simulink model "Microgrid_6DGs"  (R2024a)
settings: Solver=VariableStepAuto  StartTime=0.0  StopTime=10  RelTol=1e-3
values from neighbouring files (symbols this model uses):
  DG = cell(1, numOfDGs)    [evaluateDesigns.m]
  K = cell(1, numDGs)    [Centralized_Controller_For_DG.m]    (also in Centralized_Controller_For_DG_with_Constraints.m; ComputePassivityForDGs.m = sdpvar(1, 3, 'full'); GetPassivityForDGs.m = sdpvar(1, 3, 'full'); Global_Controller_Synthesis.m = cell(N, N))
  Line = cell(1, numOfLines)    [evaluateDesigns.m]
  numOfDGs = size(B_il,1)    [OptimizeMGparameters.m]    (also in OptimizepValsMethod1.m; centralizedCodesign.m; centralizedCodesignFeasibility.m; centralizedLocalControlDesign-Mohammad’s Laptop.m)
  V_ref = 48    [Global_Controller_Synthesis.m]
undefined symbols (not defined in the file or in its folder): change_reference, PlugIn, PlugOut, V_nom, V_ref1, V_ref2
libraries: spsSeriesRLCBranchLib x48, spsCurrentMeasurementLib x12, simulink x6, spsIdealSwitchLib x6, spsStairGeneratorLib x6, spsControlledCurrentSourceLib x6, spsDCVoltageSourceLib x6, spsDiodeLib x6, spsIGBTLib x6, spsVoltageMeasurementLib x6, spspowerguiLib x1
(part 2 of 2)

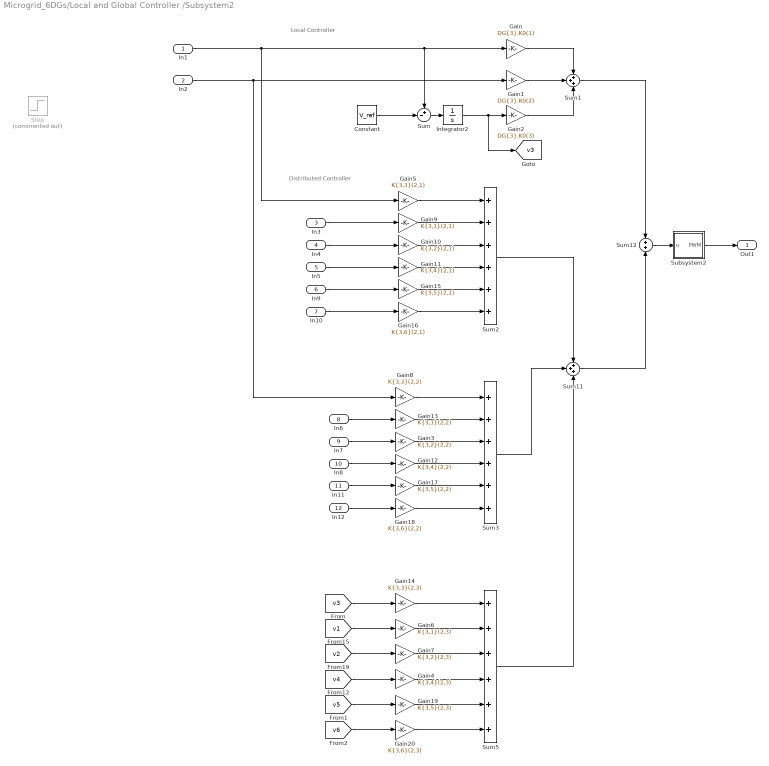
== system Microgrid_6DGs/Local and Global Controller /Subsystem2 ==
  note: Distributed Controller
  note: Local Controller
  In1 : Inport
  In2 : Inport  Port=2
  In3 : Inport  Port=3
  In4 : Inport  Port=4
  In5 : Inport  Port=5
  In9 : Inport  Port=6
  In10 : Inport  Port=7
  In6 : Inport  Port=8
  In7 : Inport  Port=9
  In8 : Inport  Port=10
  In11 : Inport  Port=11
  In12 : Inport  Port=12
  Constant : Constant  Value=V_ref
  Gain : Gain  Gain=DG{3}.K0(1)
  Gain1 : Gain  Gain=DG{3}.K0(2)
  Gain10 : Gain  Gain=K{3,2}(2,1)
  Gain11 : Gain  Gain=K{3,4}(2,1)
  Gain12 : Gain  Gain=K{3,4}(2,2)
  Gain13 : Gain  Gain=K{3,1}(2,2)
  Gain14 : Gain  Gain=K{3,3}(2,3)
  Gain15 : Gain  Gain=K{3,5}(2,1)
  Gain16 : Gain  Gain=K{3,6}(2,1)
  Gain17 : Gain  Gain=K{3,5}(2,2)
  Gain18 : Gain  Gain=K{3,6}(2,2)
  Gain19 : Gain  Gain=K{3,5}(2,3)
  Gain2 : Gain  Gain=DG{3}.K0(3)
  Gain20 : Gain  Gain=K{3,6}(2,3)
  Gain3 : Gain  Gain=K{3,2}(2,2)
  Gain4 : Gain  Gain=K{3,4}(2,3)
  Gain5 : Gain  Gain=K{3,3}(2,1)
  Gain6 : Gain  Gain=K{3,1}(2,3)
  Gain7 : Gain  Gain=K{3,2}(2,3)
  Gain8 : Gain  Gain=K{3,3}(2,2)
  Gain9 : Gain  Gain=K{3,1}(2,1)
  Integrator2 : Integrator
  Step : Step  Commented=on  Time=change_reference  Before=V_ref1  After=V_ref2  SampleTime=0
  Subsystem2 : Subsystem
      mask Display: disp('PWM')
  Sum : Sum  Inputs=+-|
  Sum1 : Sum  Inputs=+++
  Sum11 : Sum  Inputs=+++
  Sum12 : Sum  Inputs=+|+
  Sum2 : Sum  Inputs=++++++
  Sum3 : Sum  Inputs=++++++
  Sum5 : Sum  Inputs=++++++
  Out1 : Outport
  tag scope: v3=global
  wires:
  Gain/1 -> Sum1/1
  Gain1/1 -> Sum1/2
  Sum1/1 -> Sum12/1
  Gain6/1 -> Sum5/2
  Gain13/1 -> Sum3/2
  Gain12/1 -> Sum3/4
  Gain7/1 -> Sum5/3
  Gain5/1 -> Sum2/1
  Gain3/1 -> Sum3/3
  Sum11/1 -> Sum12/2
  Gain4/1 -> Sum5/4
  In4/1 -> Gain10/1
  [v2] -> Gain7/1
  In3/1 -> Gain9/1
  [v1] -> Gain6/1
  In6/1 -> Gain13/1
  [v4] -> Gain4/1
  In8/1 -> Gain12/1
  Gain10/1 -> Sum2/3
  In7/1 -> Gain3/1
  In5/1 -> Gain11/1
  Gain14/1 -> Sum5/1
  Gain11/1 -> Sum2/4
  Gain9/1 -> Sum2/2
  Gain8/1 -> Sum3/1
  [v3] -> Gain14/1
  Sum2/1 -> Sum11/1
  Sum3/1 -> Sum11/2
  Sum5/1 -> Sum11/3
  Sum/1 -> Integrator2/1
  In2/1 -> Gain1/1, Gain8/1
  In1/1 -> Gain/1, Sum/1, Gain5/1
  Sum12/1 -> Subsystem2/1(u)
  Subsystem2/1(PWM) -> Out1/1
  Constant/1 -> Sum/2
  Gain15/1 -> Sum2/5
  Gain16/1 -> Sum2/6
  In9/1 -> Gain15/1
  In10/1 -> Gain16/1
  Gain17/1 -> Sum3/5
  In11/1 -> Gain17/1
  Gain18/1 -> Sum3/6
  In12/1 -> Gain18/1
  Gain19/1 -> Sum5/5
  Gain20/1 -> Sum5/6
  [v5] -> Gain19/1
  [v6] -> Gain20/1
  Gain2/1 -> Sum1/3
  Integrator2/1 -> [v3], Gain2/1

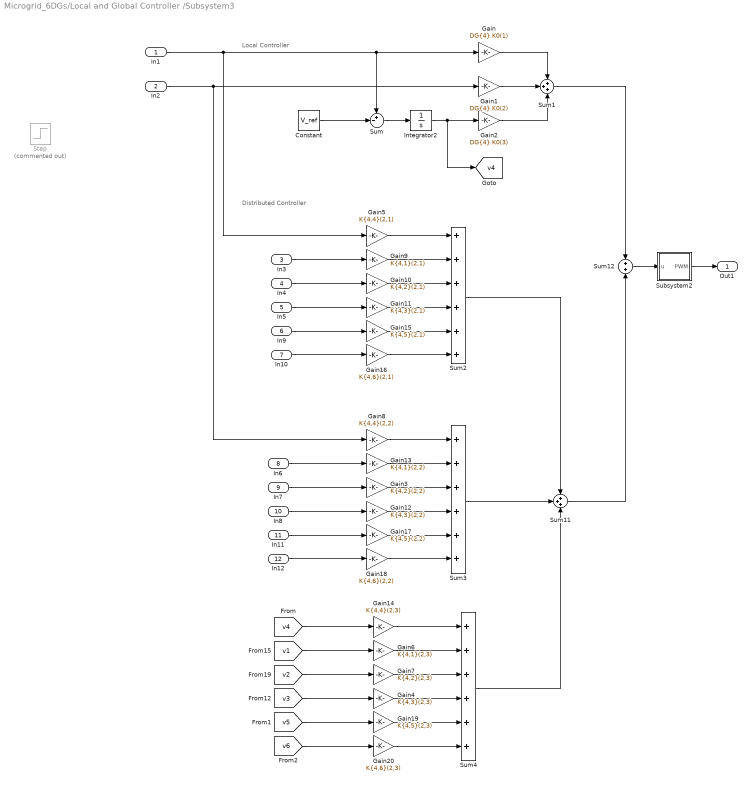
== system Microgrid_6DGs/Local and Global Controller /Subsystem3 ==
  note: Distributed Controller
  note: Local Controller
  In1 : Inport
  In2 : Inport  Port=2
  In3 : Inport  Port=3
  In4 : Inport  Port=4
  In5 : Inport  Port=5
  In9 : Inport  Port=6
  In10 : Inport  Port=7
  In6 : Inport  Port=8
  In7 : Inport  Port=9
  In8 : Inport  Port=10
  In11 : Inport  Port=11
  In12 : Inport  Port=12
  Constant : Constant  Value=V_ref
  Gain : Gain  Gain=DG{4}.K0(1)
  Gain1 : Gain  Gain=DG{4}.K0(2)
  Gain10 : Gain  Gain=K{4,2}(2,1)
  Gain11 : Gain  Gain=K{4,3}(2,1)
  Gain12 : Gain  Gain=K{4,3}(2,2)
  Gain13 : Gain  Gain=K{4,1}(2,2)
  Gain14 : Gain  Gain=K{4,4}(2,3)
  Gain15 : Gain  Gain=K{4,5}(2,1)
  Gain16 : Gain  Gain=K{4,6}(2,1)
  Gain17 : Gain  Gain=K{4,5}(2,2)
  Gain18 : Gain  Gain=K{4,6}(2,2)
  Gain19 : Gain  Gain=K{4,5}(2,3)
  Gain2 : Gain  Gain=DG{4}.K0(3)
  Gain20 : Gain  Gain=K{4,6}(2,3)
  Gain3 : Gain  Gain=K{4,2}(2,2)
  Gain4 : Gain  Gain=K{4,3}(2,3)
  Gain5 : Gain  Gain=K{4,4}(2,1)
  Gain6 : Gain  Gain=K{4,1}(2,3)
  Gain7 : Gain  Gain=K{4,2}(2,3)
  Gain8 : Gain  Gain=K{4,4}(2,2)
  Gain9 : Gain  Gain=K{4,1}(2,1)
  Integrator2 : Integrator
  Step : Step  Commented=on  Time=change_reference  Before=V_ref1  After=V_ref2  SampleTime=0
  Subsystem2 : Subsystem
      mask Display: disp('PWM')
  Sum : Sum  Inputs=+-|
  Sum1 : Sum  Inputs=+++
  Sum11 : Sum  Inputs=+++
  Sum12 : Sum  Inputs=+|+
  Sum2 : Sum  Inputs=++++++
  Sum3 : Sum  Inputs=++++++
  Sum4 : Sum  Inputs=++++++
  Out1 : Outport
  tag scope: v4=global
  wires:
  Sum1/1 -> Sum12/1
  Gain1/1 -> Sum1/2
  Gain/1 -> Sum1/1
  Gain6/1 -> Sum4/2
  Gain13/1 -> Sum3/2
  Gain12/1 -> Sum3/4
  Gain7/1 -> Sum4/3
  Gain5/1 -> Sum2/1
  Gain3/1 -> Sum3/3
  Sum11/1 -> Sum12/2
  Gain4/1 -> Sum4/4
  In4/1 -> Gain10/1
  [v2] -> Gain7/1
  In3/1 -> Gain9/1
  [v1] -> Gain6/1
  In6/1 -> Gain13/1
  [v3] -> Gain4/1
  In8/1 -> Gain12/1
  Gain10/1 -> Sum2/3
  In7/1 -> Gain3/1
  In5/1 -> Gain11/1
  Gain14/1 -> Sum4/1
  Gain11/1 -> Sum2/4
  Gain9/1 -> Sum2/2
  Gain8/1 -> Sum3/1
  [v4] -> Gain14/1
  Sum2/1 -> Sum11/1
  Sum3/1 -> Sum11/2
  Sum4/1 -> Sum11/3
  Sum/1 -> Integrator2/1
  In2/1 -> Gain1/1, Gain8/1
  In1/1 -> Gain/1, Sum/1, Gain5/1
  Sum12/1 -> Subsystem2/1(u)
  Subsystem2/1(PWM) -> Out1/1
  Constant/1 -> Sum/2
  Gain15/1 -> Sum2/5
  In9/1 -> Gain15/1
  Gain16/1 -> Sum2/6
  In10/1 -> Gain16/1
  Gain17/1 -> Sum3/5
  Gain18/1 -> Sum3/6
  In11/1 -> Gain17/1
  In12/1 -> Gain18/1
  Gain19/1 -> Sum4/5
  [v5] -> Gain19/1
  Gain20/1 -> Sum4/6
  [v6] -> Gain20/1
  Gain2/1 -> Sum1/3
  Integrator2/1 -> [v4], Gain2/1

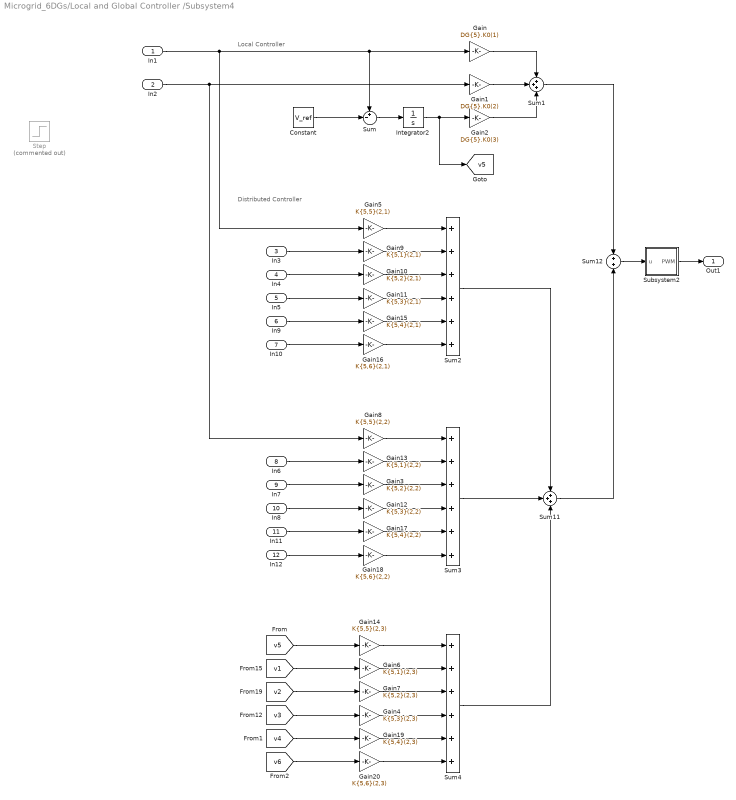
== system Microgrid_6DGs/Local and Global Controller /Subsystem4 ==
  note: Local Controller
  note: Distributed Controller
  In1 : Inport
  In2 : Inport  Port=2
  In3 : Inport  Port=3
  In4 : Inport  Port=4
  In5 : Inport  Port=5
  In9 : Inport  Port=6
  In10 : Inport  Port=7
  In6 : Inport  Port=8
  In7 : Inport  Port=9
  In8 : Inport  Port=10
  In11 : Inport  Port=11
  In12 : Inport  Port=12
  Constant : Constant  Value=V_ref
  Gain : Gain  Gain=DG{5}.K0(1)
  Gain1 : Gain  Gain=DG{5}.K0(2)
  Gain10 : Gain  Gain=K{5,2}(2,1)
  Gain11 : Gain  Gain=K{5,3}(2,1)
  Gain12 : Gain  Gain=K{5,3}(2,2)
  Gain13 : Gain  Gain=K{5,1}(2,2)
  Gain14 : Gain  Gain=K{5,5}(2,3)
  Gain15 : Gain  Gain=K{5,4}(2,1)
  Gain16 : Gain  Gain=K{5,6}(2,1)
  Gain17 : Gain  Gain=K{5,4}(2,2)
  Gain18 : Gain  Gain=K{5,6}(2,2)
  Gain19 : Gain  Gain=K{5,4}(2,3)
  Gain2 : Gain  Gain=DG{5}.K0(3)
  Gain20 : Gain  Gain=K{5,6}(2,3)
  Gain3 : Gain  Gain=K{5,2}(2,2)
  Gain4 : Gain  Gain=K{5,3}(2,3)
  Gain5 : Gain  Gain=K{5,5}(2,1)
  Gain6 : Gain  Gain=K{5,1}(2,3)
  Gain7 : Gain  Gain=K{5,2}(2,3)
  Gain8 : Gain  Gain=K{5,5}(2,2)
  Gain9 : Gain  Gain=K{5,1}(2,1)
  Integrator2 : Integrator
  Step : Step  Commented=on  Time=change_reference  Before=V_ref1  After=V_ref2  SampleTime=0
  Subsystem2 : Subsystem
      mask Display: disp('PWM')
  Sum : Sum  Inputs=+-|
  Sum1 : Sum  Inputs=+++
  Sum11 : Sum  Inputs=+++
  Sum12 : Sum  Inputs=+|+
  Sum2 : Sum  Inputs=++++++
  Sum3 : Sum  Inputs=++++++
  Sum4 : Sum  Inputs=++++++
  Out1 : Outport
  tag scope: v5=global
  wires:
  Constant/1 -> Sum/2
  Subsystem2/1(PWM) -> Out1/1
  Sum12/1 -> Subsystem2/1(u)
  In1/1 -> Gain5/1, Sum/1, Gain/1
  In2/1 -> Gain8/1, Gain1/1
  Sum/1 -> Integrator2/1
  Sum4/1 -> Sum11/3
  Sum3/1 -> Sum11/2
  Sum2/1 -> Sum11/1
  [v5] -> Gain14/1
  Gain8/1 -> Sum3/1
  Gain9/1 -> Sum2/2
  Gain11/1 -> Sum2/4
  Gain14/1 -> Sum4/1
  In5/1 -> Gain11/1
  In7/1 -> Gain3/1
  Gain10/1 -> Sum2/3
  In8/1 -> Gain12/1
  [v3] -> Gain4/1
  In6/1 -> Gain13/1
  [v1] -> Gain6/1
  In3/1 -> Gain9/1
  [v2] -> Gain7/1
  In4/1 -> Gain10/1
  Gain4/1 -> Sum4/4
  Sum11/1 -> Sum12/2
  Gain3/1 -> Sum3/3
  Gain5/1 -> Sum2/1
  Gain7/1 -> Sum4/3
  Gain12/1 -> Sum3/4
  Gain13/1 -> Sum3/2
  Gain6/1 -> Sum4/2
  Gain/1 -> Sum1/1
  Gain1/1 -> Sum1/2
  Sum1/1 -> Sum12/1
  Gain15/1 -> Sum2/5
  Gain16/1 -> Sum2/6
  In9/1 -> Gain15/1
  In10/1 -> Gain16/1
  Gain17/1 -> Sum3/5
  In11/1 -> Gain17/1
  Gain18/1 -> Sum3/6
  In12/1 -> Gain18/1
  Gain19/1 -> Sum4/5
  Gain20/1 -> Sum4/6
  [v4] -> Gain19/1
  [v6] -> Gain20/1
  Gain2/1 -> Sum1/3
  Integrator2/1 -> Gain2/1, [v5]

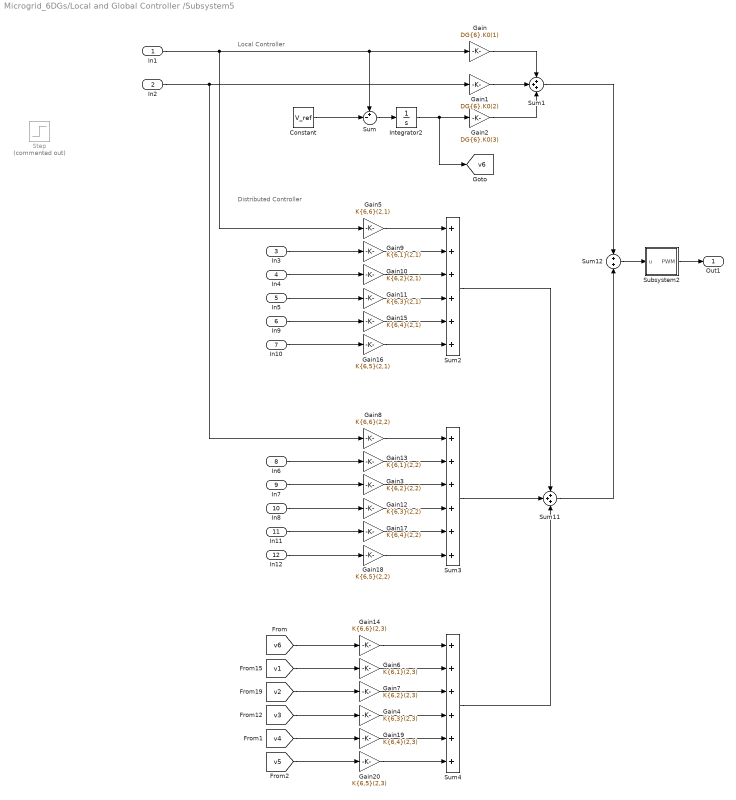
== system Microgrid_6DGs/Local and Global Controller /Subsystem5 ==
  note: Distributed Controller
  note: Local Controller
  In1 : Inport
  In2 : Inport  Port=2
  In3 : Inport  Port=3
  In4 : Inport  Port=4
  In5 : Inport  Port=5
  In9 : Inport  Port=6
  In10 : Inport  Port=7
  In6 : Inport  Port=8
  In7 : Inport  Port=9
  In8 : Inport  Port=10
  In11 : Inport  Port=11
  In12 : Inport  Port=12
  Constant : Constant  Value=V_ref
  Gain : Gain  Gain=DG{6}.K0(1)
  Gain1 : Gain  Gain=DG{6}.K0(2)
  Gain10 : Gain  Gain=K{6,2}(2,1)
  Gain11 : Gain  Gain=K{6,3}(2,1)
  Gain12 : Gain  Gain=K{6,3}(2,2)
  Gain13 : Gain  Gain=K{6,1}(2,2)
  Gain14 : Gain  Gain=K{6,6}(2,3)
  Gain15 : Gain  Gain=K{6,4}(2,1)
  Gain16 : Gain  Gain=K{6,5}(2,1)
  Gain17 : Gain  Gain=K{6,4}(2,2)
  Gain18 : Gain  Gain=K{6,5}(2,2)
  Gain19 : Gain  Gain=K{6,4}(2,3)
  Gain2 : Gain  Gain=DG{6}.K0(3)
  Gain20 : Gain  Gain=K{6,5}(2,3)
  Gain3 : Gain  Gain=K{6,2}(2,2)
  Gain4 : Gain  Gain=K{6,3}(2,3)
  Gain5 : Gain  Gain=K{6,6}(2,1)
  Gain6 : Gain  Gain=K{6,1}(2,3)
  Gain7 : Gain  Gain=K{6,2}(2,3)
  Gain8 : Gain  Gain=K{6,6}(2,2)
  Gain9 : Gain  Gain=K{6,1}(2,1)
  Integrator2 : Integrator
  Step : Step  Commented=on  Time=change_reference  Before=V_ref1  After=V_ref2  SampleTime=0
  Subsystem2 : Subsystem
      mask Display: disp('PWM')
  Sum : Sum  Inputs=+-|
  Sum1 : Sum  Inputs=+++
  Sum11 : Sum  Inputs=+++
  Sum12 : Sum  Inputs=+|+
  Sum2 : Sum  Inputs=++++++
  Sum3 : Sum  Inputs=++++++
  Sum4 : Sum  Inputs=++++++
  Out1 : Outport
  tag scope: v6=global
  wires:
  [v5] -> Gain20/1
  [v4] -> Gain19/1
  Gain20/1 -> Sum4/6
  Gain19/1 -> Sum4/5
  In12/1 -> Gain18/1
  Gain18/1 -> Sum3/6
  In11/1 -> Gain17/1
  Gain17/1 -> Sum3/5
  In10/1 -> Gain16/1
  In9/1 -> Gain15/1
  Gain16/1 -> Sum2/6
  Gain15/1 -> Sum2/5
  Sum1/1 -> Sum12/1
  Gain1/1 -> Sum1/2
  Gain/1 -> Sum1/1
  Gain6/1 -> Sum4/2
  Gain13/1 -> Sum3/2
  Gain12/1 -> Sum3/4
  Gain7/1 -> Sum4/3
  Gain5/1 -> Sum2/1
  Gain3/1 -> Sum3/3
  Sum11/1 -> Sum12/2
  Gain4/1 -> Sum4/4
  In4/1 -> Gain10/1
  [v2] -> Gain7/1
  In3/1 -> Gain9/1
  [v1] -> Gain6/1
  In6/1 -> Gain13/1
  [v3] -> Gain4/1
  In8/1 -> Gain12/1
  Gain10/1 -> Sum2/3
  In7/1 -> Gain3/1
  In5/1 -> Gain11/1
  Gain14/1 -> Sum4/1
  Gain11/1 -> Sum2/4
  Gain9/1 -> Sum2/2
  Gain8/1 -> Sum3/1
  [v6] -> Gain14/1
  Sum2/1 -> Sum11/1
  Sum3/1 -> Sum11/2
  Sum4/1 -> Sum11/3
  Sum/1 -> Integrator2/1
  In2/1 -> Gain1/1, Gain8/1
  In1/1 -> Gain/1, Sum/1, Gain5/1
  Sum12/1 -> Subsystem2/1(u)
  Subsystem2/1(PWM) -> Out1/1
  Constant/1 -> Sum/2
  Gain2/1 -> Sum1/3
  Integrator2/1 -> [v6], Gain2/1

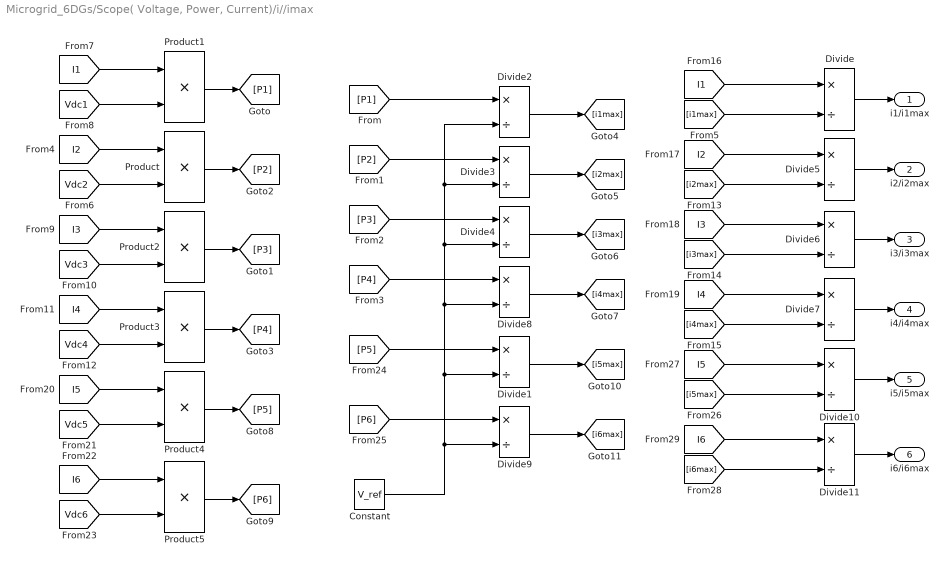
== system Microgrid_6DGs/Scope( Voltage, Power, Current)/i//imax ==
  Constant : Constant  Value=V_ref
  Divide{,1..11} (12 alike) : Product  Inputs=*/
  Product{,1..5} (6 alike) : Product
  i1/i1max : Outport  VectorParamsAs1DForOutWhenUnconnected=off
  i2/i2max : Outport  Port=2  VectorParamsAs1DForOutWhenUnconnected=off
  i3/i3max : Outport  Port=3  VectorParamsAs1DForOutWhenUnconnected=off
  i4/i4max : Outport  Port=4  VectorParamsAs1DForOutWhenUnconnected=off
  i5/i5max : Outport  Port=5  VectorParamsAs1DForOutWhenUnconnected=off
  i6/i6max : Outport  Port=6  VectorParamsAs1DForOutWhenUnconnected=off
  wires:
  Divide/1 -> i1/i1max/1
  Divide5/1 -> i2/i2max/1
  Divide6/1 -> i3/i3max/1
  Divide7/1 -> i4/i4max/1
  [Vdc3] -> Product2/2
  [Vdc1] -> Product1/2
  [Vdc2] -> Product/2
  [I1] -> Product1/1
  [I2] -> Product/1
  [Vdc4] -> Product3/2
  [I4] -> Product3/1
  [I3] -> Product2/1
  Product1/1 -> [P1]
  Product2/1 -> [P3]
  Product/1 -> [P2]
  Product3/1 -> [P4]
  [P1] -> Divide2/1
  [P2] -> Divide3/1
  [P3] -> Divide4/1
  [P4] -> Divide8/1
  Constant/1 -> Divide9/2, Divide1/2, Divide8/2, Divide4/2, Divide3/2, Divide2/2
  Divide8/1 -> [i4max]
  Divide4/1 -> [i3max]
  Divide3/1 -> [i2max]
  Divide2/1 -> [i1max]
  [i1max] -> Divide/2
  [i2max] -> Divide5/2
  [i3max] -> Divide6/2
  [i4max] -> Divide7/2
  [I1] -> Divide/1
  [I2] -> Divide5/1
  [I3] -> Divide6/1
  [I4] -> Divide7/1
  Product4/1 -> [P5]
  [I5] -> Product4/1
  [Vdc5] -> Product4/2
  [Vdc6] -> Product5/2
  [I6] -> Product5/1
  Product5/1 -> [P6]
  [P5] -> Divide1/1
  [P6] -> Divide9/1
  Divide1/1 -> [i5max]
  Divide9/1 -> [i6max]
  [I5] -> Divide10/1
  [i5max] -> Divide10/2
  Divide10/1 -> i5/i5max/1
  Divide11/1 -> i6/i6max/1
  [i6max] -> Divide11/2
  [I6] -> Divide11/1

== system Microgrid_6DGs/Subsystem/Breaker3 ==
  Ideal Switch : spsIdealSwitchLib/Ideal Switch  Ron=0.001  Lon=0  IC=0  Rs=1e5  Cs=inf  Measurements=on
  Stair Generator : spsStairGeneratorLib/Stair Generator  t=[0,PlugOut,PlugIn]  e=[1, 0, 1]  Ts=0
  DG3 : PMIOPort  Side=Left
  + : PMIOPort  Port=2  Side=Right
  wires:
  Stair Generator/1 -> Ideal Switch/1
  connections:
  Ideal Switch/LConn1 -- DG3/RConn1
  Ideal Switch/RConn1 -- +/RConn1

== system Microgrid_6DGs/Subsystem1/Breaker1 ==
  Ideal Switch : spsIdealSwitchLib/Ideal Switch  Ron=0.001  Lon=0  IC=0  Rs=1e5  Cs=inf  Measurements=on
  Stair Generator : spsStairGeneratorLib/Stair Generator  t=[0,PlugOut,PlugIn]  e=[1, 0, 1]  Ts=0
  DG1 : PMIOPort  Side=Left
  + : PMIOPort  Port=2  Side=Right
  wires:
  Stair Generator/1 -> Ideal Switch/1
  connections:
  Ideal Switch/LConn1 -- DG1/RConn1
  Ideal Switch/RConn1 -- +/RConn1

== system Microgrid_6DGs/Subsystem2/Breaker1 ==
  Ideal Switch : spsIdealSwitchLib/Ideal Switch  Ron=0.001  Lon=0  IC=0  Rs=1e5  Cs=inf  Measurements=on
  Stair Generator : spsStairGeneratorLib/Stair Generator  t=[0,PlugOut,PlugIn]  e=[1, 0, 1]  Ts=0
  DG1 : PMIOPort  Side=Left
  + : PMIOPort  Port=2  Side=Right
  wires:
  Stair Generator/1 -> Ideal Switch/1
  connections:
  Ideal Switch/RConn1 -- +/RConn1
  Ideal Switch/LConn1 -- DG1/RConn1

== system Microgrid_6DGs/Subsystem4/Breaker1 ==
  Ideal Switch : spsIdealSwitchLib/Ideal Switch  Ron=0.001  Lon=0  IC=0  Rs=1e5  Cs=inf  Measurements=on
  Stair Generator : spsStairGeneratorLib/Stair Generator  t=[0,PlugOut,PlugIn]  e=[1, 0, 1]  Ts=0
  DG1 : PMIOPort  Side=Left
  + : PMIOPort  Port=2  Side=Right
  wires:
  Stair Generator/1 -> Ideal Switch/1
  connections:
  Ideal Switch/RConn1 -- +/RConn1
  Ideal Switch/LConn1 -- DG1/RConn1

== system Microgrid_6DGs/Subsystem5/Breaker ==
  Ideal Switch : spsIdealSwitchLib/Ideal Switch  Ron=0.001  Lon=0  IC=0  Rs=1e5  Cs=inf  Measurements=on
  Stair Generator : spsStairGeneratorLib/Stair Generator  t=[0,PlugOut,PlugIn]  e=[1, 0, 1]  Ts=0
  DG2 : PMIOPort  Side=Left
  + : PMIOPort  Port=2  Side=Right
  wires:
  Stair Generator/1 -> Ideal Switch/1
  connections:
  Ideal Switch/LConn1 -- DG2/RConn1
  Ideal Switch/RConn1 -- +/RConn1

== system Microgrid_6DGs/Subsystem6/Breaker ==
  Ideal Switch : spsIdealSwitchLib/Ideal Switch  Ron=0.001  Lon=0  IC=0  Rs=1e5  Cs=inf  Measurements=on
  Stair Generator : spsStairGeneratorLib/Stair Generator  t=[0,PlugOut,PlugIn]  e=[1, 0, 1]  Ts=0
  DG4 : PMIOPort  Side=Left
  + : PMIOPort  Port=2  Side=Right
  wires:
  Stair Generator/1 -> Ideal Switch/1
  connections:
  Ideal Switch/LConn1 -- DG4/RConn1
  Ideal Switch/RConn1 -- +/RConn1

== system Microgrid_6DGs/Local and Global Controller /Subsystem/Subsystem2 ==
  u : Inport
  0.05 : Gain
  Relational Operator : RelationalOperator  OutDataTypeStr=boolean  InputSameDT=off
  Scope : Scope  NumInputPorts=2
  Scope2 : Scope
  Triangle1 : simulink/Sources/Repeating Sequence  rep_seq_t=[0 40e-5 80e-5]  rep_seq_y=[0 1 0]
  PWM : Outport
  wires:
  0.05/1 -> Relational Operator/1, Scope/1
  Triangle1/1 -> Relational Operator/2, Scope/2
  u/1 -> 0.05/1
  Relational Operator/1 -> PWM/1, Scope2/1

== system Microgrid_6DGs/Local and Global Controller /Subsystem1/Subsystem2 ==
  u : Inport
  0.05 : Gain
  Relational Operator : RelationalOperator  OutDataTypeStr=boolean  InputSameDT=off
  Scope : Scope  NumInputPorts=2
  Scope2 : Scope
  Triangle1 : simulink/Sources/Repeating Sequence  rep_seq_t=[0 40e-5 80e-5]  rep_seq_y=[0 1 0]
  PWM : Outport
  wires:
  0.05/1 -> Relational Operator/1, Scope/1
  Triangle1/1 -> Relational Operator/2, Scope/2
  u/1 -> 0.05/1
  Relational Operator/1 -> PWM/1, Scope2/1

== system Microgrid_6DGs/Local and Global Controller /Subsystem2/Subsystem2 ==
  u : Inport
  0.05 : Gain
  Relational Operator : RelationalOperator  OutDataTypeStr=boolean  InputSameDT=off
  Scope : Scope  NumInputPorts=2
  Scope2 : Scope
  Triangle1 : simulink/Sources/Repeating Sequence  rep_seq_t=[0 40e-5 80e-5]  rep_seq_y=[0 1 0]
  PWM : Outport
  wires:
  0.05/1 -> Relational Operator/1, Scope/1
  Triangle1/1 -> Relational Operator/2, Scope/2
  u/1 -> 0.05/1
  Relational Operator/1 -> PWM/1, Scope2/1

== system Microgrid_6DGs/Local and Global Controller /Subsystem3/Subsystem2 ==
  u : Inport
  0.05 : Gain
  Relational Operator : RelationalOperator  OutDataTypeStr=boolean  InputSameDT=off
  Scope : Scope  NumInputPorts=2
  Scope2 : Scope
  Triangle1 : simulink/Sources/Repeating Sequence  rep_seq_t=[0 40e-5 80e-5]  rep_seq_y=[0 1 0]
  PWM : Outport
  wires:
  0.05/1 -> Relational Operator/1, Scope/1
  Triangle1/1 -> Relational Operator/2, Scope/2
  u/1 -> 0.05/1
  Relational Operator/1 -> PWM/1, Scope2/1

== system Microgrid_6DGs/Local and Global Controller /Subsystem4/Subsystem2 ==
  u : Inport
  0.05 : Gain
  Relational Operator : RelationalOperator  OutDataTypeStr=boolean  InputSameDT=off
  Scope : Scope  NumInputPorts=2
  Scope2 : Scope
  Triangle1 : simulink/Sources/Repeating Sequence  rep_seq_t=[0 40e-5 80e-5]  rep_seq_y=[0 1 0]
  PWM : Outport
  wires:
  Relational Operator/1 -> Scope2/1, PWM/1
  u/1 -> 0.05/1
  Triangle1/1 -> Scope/2, Relational Operator/2
  0.05/1 -> Scope/1, Relational Operator/1

== system Microgrid_6DGs/Local and Global Controller /Subsystem5/Subsystem2 ==
  u : Inport
  0.05 : Gain
  Relational Operator : RelationalOperator  OutDataTypeStr=boolean  InputSameDT=off
  Scope : Scope  NumInputPorts=2
  Scope2 : Scope
  Triangle1 : simulink/Sources/Repeating Sequence  rep_seq_t=[0 40e-5 80e-5]  rep_seq_y=[0 1 0]
  PWM : Outport
  wires:
  0.05/1 -> Relational Operator/1, Scope/1
  Triangle1/1 -> Relational Operator/2, Scope/2
  u/1 -> 0.05/1
  Relational Operator/1 -> PWM/1, Scope2/1
